simulink model "mae_forced"  (R2021b)
settings: Solver=VariableStepAuto  StartTime=0.0  StopTime=10  MaxStep=0.005  RelTol=1e-3  AbsTol=1e-3  EnableMultiTasking=on
PostLoadFcn:
  | m = 3.600;     % kg
  | k = 400;    % N/m
  | b = 10;      % Ns/m
CloseFcn:
  | try,close(h1_ssc_mass_spring_damper_sl_dbl),end
  | clear h1_ssc_mass_spring_damper_sl_dbl
  | 
  | clear simlog_ssc_mass_spring_damper_sl_dbl
  | clear logsout_ssc_mass_spring_damper_sl_dbl
Description:
  | Double Mass-Spring-Damper in Simulink(R) and Simscape(TM)
settings Model: Creator=The MathWorks, Inc.  LastModifiedBy=Admin
settings SolverCC: AutoScaleAbsTol=off  AlgebraicLoopSolver=TrustRegion
settings DataIOCC: SaveFormat=Array  ReturnWorkspaceOutputs=off  SignalLoggingName=logsout_ssc_mass_spring_damper_sl_dbl
settings OptimizationCC: LifeSpan=inf
settings DebuggingCC: SolverPrmCheckMsg=warning  AllowSymbolicDim=off  PregeneratedLibrarySubsystemCodeDiagnostic=none  SFUnexpectedBacktrackingDiag=warning  SFNoUnconditionalDefaultTransitionDiag=warning  SFExecutionAtInitializationDiag=none  SFMachineParentedDataDiag=warning  ArithmeticOperatorsInVariantConditions=warning
settings HardwareCC: ProdBitPerPointer=32  ProdBitPerSizeT=32  ProdBitPerPtrDiffT=32  ProdLargestAtomicFloat=None  ProdIntDivRoundTo=Undefined  ProdEndianess=Unspecified  ProdWordSize=32  ProdHWDeviceType=32-bit Generic
settings ModelReferenceCC: PropagateSignalLabelsOutOfModel=off
settings SFSimCC: SimUseLocalCustomCode=off  CustomCodeUndefinedFunction=UseInterfaceOnly
settings RTWCC: RTWUseLocalCustomCode=off
settings CodeAppCC: StateflowObjectComments=on
settings GRTTargetCC: TargetLangStandard=C89/C90 (ANSI)
settings ConfigComp: CovMetricSettings=dw  CovSaveCumulativeToWorkspaceVar=on  CovSaveSingleToWorkspaceVar=on  CovExternalEMLEnable=off  CovSFcnEnable=off
settings SimscapeCC: SimscapeLogType=all  SimscapeLogSimulationStatistics=on  SimscapeLogName=simlog_ssc_mass_spring_damper_sl_dbl  SimscapeLogDataHistory=10000

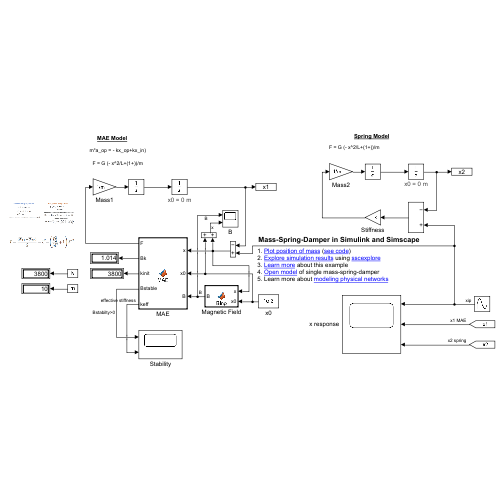
[thumbnail: Simulink's stored preview of the top-level diagram]
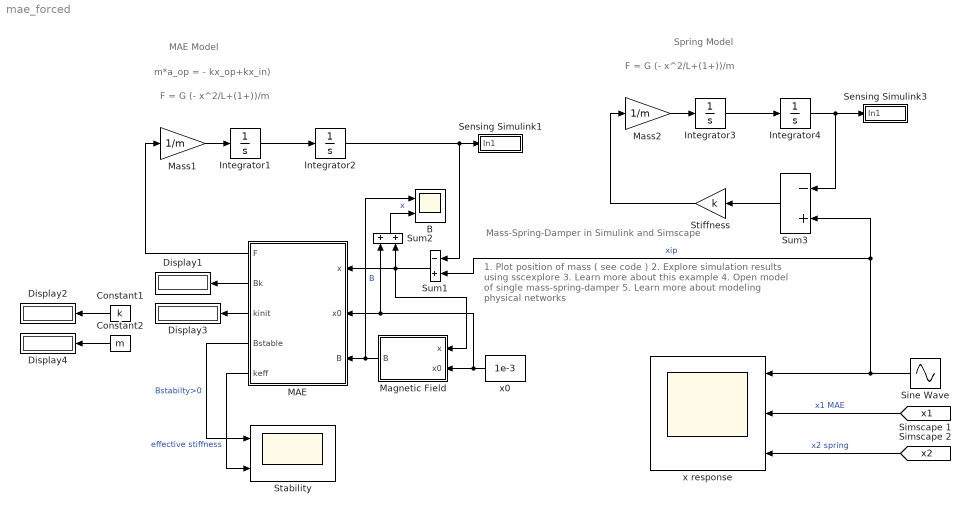
== system mae_forced ==
  note: 1. Plot position of mass ( see code )
      | 2. Explore simulation results using sscexplore
      | 3. Learn more about this example
      | 4. Open model of single mass-spring-damper
      | 5. Learn more about modeling physical networks
  note: Mass-Spring-Damper in Simulink and Simscape
  note: MAE Model
  note: m*a_op = - kx_op+kx_in)
  note: F = G (- x^2/L+(1+))/m
  note: F = G (- x^2/L+(1+))/m
  note: Spring Model
  B : Scope  NumInputPorts=2
  Constant1 : Constant  Value=k
  Constant2 : Constant  Value=m
  Display{1..4} (4 alike) : Display
  Integrator{1..4} (4 alike) : Integrator
      Integrator2 settings: AttributesFormatString=x0 = %<InitialCondition> m
      Integrator4 settings: AttributesFormatString=x0 = %<InitialCondition> m
  MAE : MATLAB Function  TreatAsAtomicUnit=on
  Magnetic Field : MATLAB Function  TreatAsAtomicUnit=on
  Mass1 : Gain  Gain=1/m  SaturateOnIntegerOverflow=on  OutDataTypeStr=Inherit: Same as input  ParamDataTypeStr=Inherit: Same as input
  Mass2 : Gain  Gain=1/m  SaturateOnIntegerOverflow=on  OutDataTypeStr=Inherit: Same as input  ParamDataTypeStr=Inherit: Same as input
  Sensing Simulink1 : Subsystem
      mask Display: disp('x1')
  Sensing Simulink3 : Subsystem
      mask Display: disp('x2')
  Sine Wave : Sin  Amplitude=1e-3  Frequency=2  SampleTime=0
  Stability : Scope  NumInputPorts=2
  Stiffness : Gain  Gain=k  SaturateOnIntegerOverflow=on  OutDataTypeStr=Inherit: Same as input  ParamDataTypeStr=Inherit: Same as input
  Sum1 : Sum  Inputs=-+  InputSameDT=on  SaturateOnIntegerOverflow=on  OutDataTypeStr=Inherit: Same as first input
  Sum2 : Sum  InputSameDT=on  SaturateOnIntegerOverflow=on  OutDataTypeStr=Inherit: Same as first input
  Sum3 : Sum  Inputs=-+  InputSameDT=on  SaturateOnIntegerOverflow=on  OutDataTypeStr=Inherit: Same as first input
  x response : Scope  NumInputPorts=3
  x0 : Constant  Value=1e-3
  wires:
  Mass1/1 -> Integrator1/1
  Integrator2/1 -> Sum1/1, Sensing Simulink1/1(In1)
  Integrator1/1 -> Integrator2/1
  MAE/2(Bk) -> Display1/1
  Constant1/1 -> Display2/1
  [x1] -> x response/2  "x1 MAE"
  MAE/4(Bstable) -> Stability/1  "Bstabilty>0"
  MAE/3(kinit) -> Display3/1
  Constant2/1 -> Display4/1
  Mass2/1 -> Integrator3/1
  Integrator3/1 -> Integrator4/1
  Stiffness/1 -> Mass2/1
  Integrator4/1 -> Sum3/1, Sensing Simulink3/1(In1)
  [x2] -> x response/3  "x2 spring"
  Magnetic Field/1(B) -> MAE/3(B), B/1  "B"
  MAE/1(F) -> Mass1/1
  Sum1/1 -> Sum2/2, MAE/1(x), Magnetic Field/1(x)
  Sine Wave/1 -> Sum1/2, Sum3/2, x response/1  "xip"
  Sum3/1 -> Stiffness/1
  MAE/5(keff) -> Stability/2  "effective stiffness"
  x0/1 -> Sum2/1, MAE/2(x0), Magnetic Field/2(x0)
  Sum2/1 -> B/2  "x"

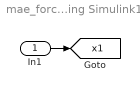
== system mae_forced/Sensing Simulink1 ==
  In1 : Inport
  tag scope: x1=global
  wires:
  In1/1 -> [x1]

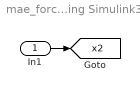
== system mae_forced/Sensing Simulink3 ==
  In1 : Inport
  tag scope: x2=global
  wires:
  In1/1 -> [x2]

== matlab function mae_forced/Magnetic Field ==
  data: x input; B output; x0 input
function B = BInp(x,x0)
G1 = 50*1e3;    c1 = 0.9;       mu1 = 1;                                
G2 = 500*1e3;   c2 = 0.1;       mu2 = 10;                               

mu0 = 1.25663706 * 1e-6;        L0 = 0.01;
Gbar = G1*c1 + G2*c2;           mubar = mu0*(mu1*c1 + mu2*c2);   
Gcap = 1/(c1/G1 + c2/G2);       mucap = mu0/(c1/mu1 + c2/mu2);

% A = L0*L0;

ld = 1 + (x+x0)/L0;                  
% Bk =  B^2/(mucap*Gbar);
% F = A*Gbar*(ld^2 - 1/ld^2 - Bk/ld^2);

Bk = ld^4-1;
if Bk>0
    B = sqrt((mucap*Gbar)*Bk);
else
    B = 0;
end

% Bstable = (ld^4-1+Gcap/Gbar)*(mucap*Gbar)/(1-mucap/mubar) - B^2;

== matlab function mae_forced/MAE ==
  data: x input; x0 input; B input; F output; Bk output; kinit output; Bstable output; keff output
function [F,Bk,kinit,Bstable,keff] = MAE(x,x0,B)

G1 = 50*1e3;    c1 = 0.9;       mu1 = 1;                                
G2 = 500*1e3;   c2 = 0.1;       mu2 = 10;                               

mu0 = 1.25663706 * 1e-6;        L0 = 0.01;
Gbar = G1*c1 + G2*c2;           mubar = mu0*(mu1*c1 + mu2*c2);   
Gcap = 1/(c1/G1 + c2/G2);       mucap = mu0/(c1/mu1 + c2/mu2);

A = L0*L0;


ld = 1 + (x+x0)/L0;                   
Bk =  B^2/(mucap*Gbar);
kinit = A*Gbar*(2 + 2)/L0;
keff = A*Gbar*2*(ld + 1/ld^3 + Bk/ld^3)/L0;

F = A*Gbar*(ld^2 - 1/ld^2 - Bk/ld^2);

Bstable = (ld^4-1+Gcap/Gbar)*(mucap*Gbar)/(1-mucap/mubar) - B^2;

end
